simulink model "controllo_op_space"  (R2024a)
settings: Solver=VariableStepAuto  StartTime=0.0  StopTime=70  RelTol=1e-3
values from neighbouring files (symbols this model uses):
  a1 = 0.5    [avvicinamentosingolaritaforza 1.m]    (also in avvicinamentosingolaritaforza.m; cubic.m = 0; dynamicmodel.m; traiettoriafperfettadefinitiva1.m)
  a2 = 0.5    [avvicinamentosingolaritaforza 1.m]    (also in avvicinamentosingolaritaforza.m; cubic.m = 3*(s_f-s_i)/delta_t^2; dynamicmodel.m; traiettoriafperfettadefinitiva1.m)
settings Model: Creator=ACER  LastModifiedBy=UTENTE
settings OptimizationCC: ReuseModelBlockBuffer=off
settings RTWCC: GPUComputeCapability=3.5

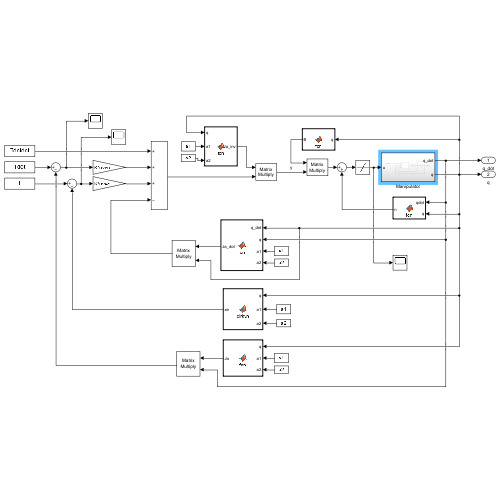
[thumbnail: Simulink's stored preview of the top-level diagram]
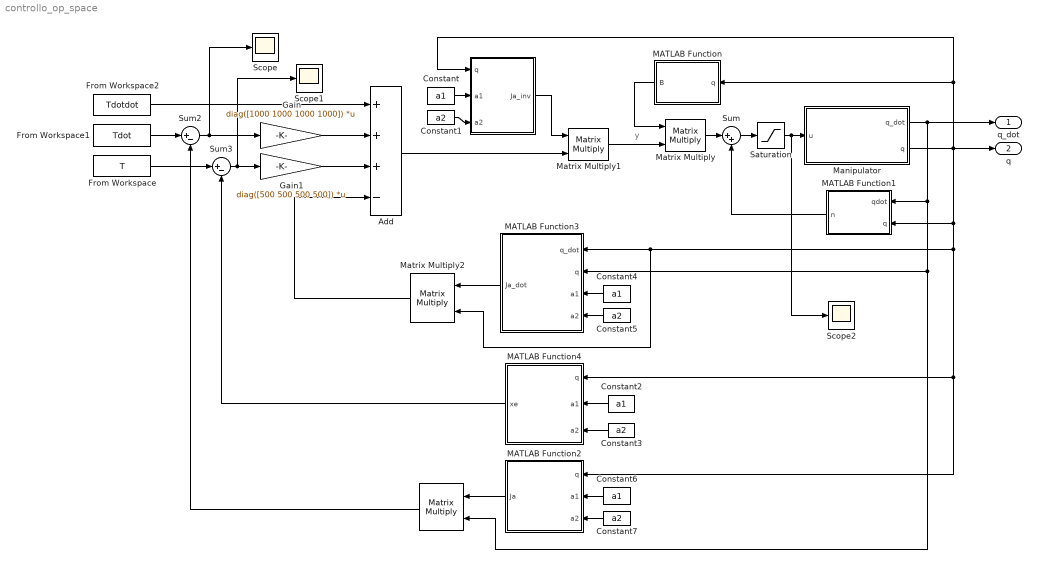
== system controllo_op_space ==
  note: y
  "  " : MATLAB Function  TreatAsAtomicUnit=on
  "   " : Product  Multiplication=Matrix(*)
  Add : Sum  Inputs=+++-
  Constant{,2,4,6} (4 alike) : Constant  Value=a1
  Constant{1,3,5,7} (4 alike) : Constant  Value=a2
  From Workspace : FromWorkspace  VariableName=T  SampleTime=0.001
  From Workspace1 : FromWorkspace  VariableName=Tdot  SampleTime=0.001
  From Workspace2 : FromWorkspace  VariableName=Tdotdot  SampleTime=0.001
  Gain : Gain  Gain=diag([1000 1000 1000 1000])  Multiplication=Matrix(K*u) (u vector)
  Gain1 : Gain  Gain=diag([500 500 500 500])  Multiplication=Matrix(K*u) (u vector)
  MATLAB Function : MATLAB Function  TreatAsAtomicUnit=on
  MATLAB Function1 : MATLAB Function  TreatAsAtomicUnit=on
  MATLAB Function2 : MATLAB Function  TreatAsAtomicUnit=on
  MATLAB Function3 : MATLAB Function  TreatAsAtomicUnit=on
  MATLAB Function4 : MATLAB Function  TreatAsAtomicUnit=on
  Manipulator : Subsystem
  Matrix Multiply : Product  Multiplication=Matrix(*)
  Matrix Multiply1 : Product  Multiplication=Matrix(*)
  Matrix Multiply2 : Product  Multiplication=Matrix(*)
  Saturation : Saturate  UpperLimit=2000  LowerLimit=-2000
  Scope : Scope
  Scope1 : Scope
  Scope2 : Scope
  Sum : Sum  Inputs=|++
  Sum2 : Sum  Inputs=|+-
  Sum3 : Sum  Inputs=|+-
  q_dot : Outport
  q : Outport  Port=2
  wires:
  MATLAB Function1/1(n) -> Sum/2
  Matrix Multiply/1 -> Sum/1
  Sum/1 -> Saturation/1
  MATLAB Function/1(B) -> Matrix Multiply/1
  Matrix Multiply1/1 -> Matrix Multiply/2
  "  "/1(Ja_inv) -> Matrix Multiply1/1
  Constant1/1 -> "  "/3(a2)
  Constant/1 -> "  "/2(a1)
  From Workspace2/1 -> Add/1
  From Workspace1/1 -> Sum2/1
  From Workspace/1 -> Sum3/1
  Sum2/1 -> Scope/1, Gain/1
  Gain/1 -> Add/2
  Sum3/1 -> Scope1/1, Gain1/1
  Gain1/1 -> Add/3
  MATLAB Function4/1(xe) -> Sum3/2
  "   "/1 -> Sum2/2
  Matrix Multiply2/1 -> Add/4
  Add/1 -> Matrix Multiply1/2
  Constant5/1 -> MATLAB Function3/4(a2)
  Constant4/1 -> MATLAB Function3/3(a1)
  Manipulator/2(q) -> q/1, MATLAB Function2/1(q), MATLAB Function4/1(q), Matrix Multiply2/2, MATLAB Function3/1(q_dot), MATLAB Function1/2(q), "  "/1(q), MATLAB Function/1(q)
  MATLAB Function3/1(Ja_dot) -> Matrix Multiply2/1
  Manipulator/1(q_dot) -> q_dot/1, "   "/2, MATLAB Function3/2(q), MATLAB Function1/1(qdot)
  MATLAB Function2/1(Ja) -> "   "/1
  Constant6/1 -> MATLAB Function2/2(a1)
  Constant7/1 -> MATLAB Function2/3(a2)
  Constant2/1 -> MATLAB Function4/2(a1)
  Constant3/1 -> MATLAB Function4/3(a2)
  Saturation/1 -> Scope2/1, Manipulator/1(u)

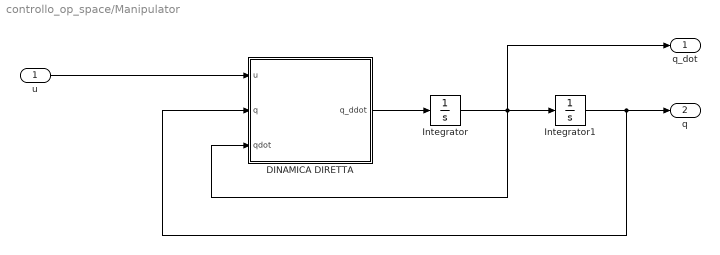
== system controllo_op_space/Manipulator ==
  u : Inport
  DINAMICA DIRETTA : MATLAB Function  TreatAsAtomicUnit=on
  Integrator : Integrator  InitialCondition=[0 0 0 0]'
  Integrator1 : Integrator  InitialCondition=[0 -pi/4 0 0]
  q_dot : Outport  VectorParamsAs1DForOutWhenUnconnected=off
  q : Outport  Port=2  VectorParamsAs1DForOutWhenUnconnected=off
  wires:
  Integrator1/1 -> q/1, DINAMICA DIRETTA/2(q)
  Integrator/1 -> q_dot/1, DINAMICA DIRETTA/3(qdot), Integrator1/1
  DINAMICA DIRETTA/1(q_ddot) -> Integrator/1
  u/1 -> DINAMICA DIRETTA/1(u)

== matlab function controllo_op_space/MATLAB Function1 ==
  data: qdot input; q input; n output
function n = fcn(qdot, q)
a1=0.5; %m
a2=0.5; %m
l1=0.25; %m
l2=0.25; %m
ml1=20; %kg
ml2=20; %kg
ml3=10; %kg
Il1=4; %kg*m^2
Il2=4; %kg*m^2
Il4=1; %kg*m^2
kr1=1;
kr2=1;
kr3=50; %rad/m
kr4 =20;
Im1=0.01; %kg*m^2
Im2=0.01; %kg*m^2
Im3=0.005; %kg*m^2
Im4=0.001; %kg*m^2
Fm1=0.00005; %N*m*s/rad
Fm2=0.00005; %N*m*s/rad
Fm3 =0.01; %N*m*s/rad
Fm4 =0.005; %N*m*s/rad
mpayload=5;

%% CALCOLO JPl JPm JOl JOm

Jp_l1=[-l1*sin(q(1)) 0 0 0;
    l1*cos(q(1)) 0 0 0;
    0 0 0 0];

Jp_l2=[-a1*sin(q(1))-l2*sin(q(1)+q(2)) -l2*sin(q(1)+q(2)) 0 0;
    a1*cos(q(1))+l2*cos(q(1)+q(2)) l2*cos(q(1)+q(2)) 0 0;
    0 0 0 0];

%poiché ml3 è nulla è inutile calcolare Jp_l3

Jp_l4=[-a1*sin(q(1))-a2*sin(q(1)+q(2)) -a2*sin(q(1)+q(2)) 0 0;
    a1*cos(q(1))+a2*cos(q(1)+q(2)) a2*cos(q(1)+q(2)) 0 0;
    0 0 -1 0];      %Jp_l4=Ja


Jo_l1=[zeros(2,4)
    1 0 0 0]; 

Jo_l2=[zeros(2,4)
    1 1 0 0];

%poiché Il3 è nullo è inutile calcolare Jo_l3

Jo_l4=[zeros(2,4)
    1 1 0 -1];       %Jo_l4=Ja;


%poiché le masse dei motori sono nulle, è inutile calcolare Jp_m 

Jo_m1=[zeros(2,4)
    kr1 0 0 0]; 

Jo_m2=[zeros(2,4)
    1 kr2 0 0];

Jo_m3=[zeros(2,4)
    1 1 kr3 0];

Jo_m4=[zeros(2,4)
    1 1 0 -kr4];  

%% CALCOLO MATRICE B (tenendo conto di braccio aumentato)
B=  ml1*(Jp_l1'*Jp_l1)+Jo_l1'*Il1*Jo_l1+Jo_m1'*Im1*Jo_m1...
    +ml2*(Jp_l2'*Jp_l2)+Jo_l2'*Il2*Jo_l2+Jo_m2'*Im2*Jo_m2...
    +Jo_m3'*Im3*Jo_m3+...
    +ml3*(Jp_l4'*Jp_l4)+Jo_l4'*Il4*Jo_l4+Jo_m4'*Im4*Jo_m4;

%% JACOBIANO DERIVATO RISPETTO A dq1 e dq2

%Jpl1 dipende solo da q1
Jpl1_dq1=[-l1*cos(q(1)) 0 0 0;
    -l1*sin(q(1)) 0 0 0;
    0 0 0 0];

Jpl2_dq1=[-a1*cos(q(1))-l2*cos(q(1)+q(2)) -l2*cos(q(1)+q(2)) 0 0;
    -a1*sin(q(1))-l2*sin(q(1)+q(2)) -l2*sin(q(1)+q(2)) 0 0;
    0 0 0 0];

Jpl2_dq2=[-a2*cos(q(1)+q(2)) -a2*cos(q(1)+q(2)) 0 0;
    -a2*sin(q(1)+q(2)) -a2*sin(q(1)+q(2)) 0 0;
    0 0 0 0];

Jpl4_dq1=[-a1*cos(q(1))-a2*cos(q(1)+q(2)) -a2*cos(q(1)+q(2)) 0 0;
    -a1*sin(q(1))-a2*sin(q(1)+q(2)) -a2*sin(q(1)+q(2)) 0 0;
    0 0 0 0];

Jpl4_dq2=[-a2*sin(q(1)+q(2)) -a2*sin(q(1)+q(2)) 0 0;
    -a2*cos(q(1)+q(2)) -a2*cos(q(1)+q(2)) 0 0;
    0 0 0 0];

%i Jo non dipendono da nessuna q

%% Calcolo matrice differenziate rispetto a dq1 dq2
dBdq1=ml1*(Jpl1_dq1'*Jp_l1+Jp_l1'*Jpl1_dq1)+ml2*(Jpl2_dq1'*Jp_l2+Jp_l2'*Jpl2_dq1)...
    +ml3*(Jpl4_dq1'*Jp_l4+Jp_l4'*Jpl4_dq1);
dBdq2=ml2*(Jpl2_dq2'*Jp_l2+Jp_l2'*Jpl2_dq2)+ml3*(Jpl4_dq2'*Jp_l4+Jp_l4'*Jpl4_dq2);

%B non dipende da q3 e q4

H=zeros(4,4,4);

%% Inizializzazione simboli cristoffel del primo tipo
for i=1:4
    for j=1:4
        for k=1:4
            H(i,j,k)=0;
        end
    end
end

%ricordiamo che B è simmetrica quindi hijk=hikj
%inoltre tutti i hiii sono nulli

H(1,1,2)=1/2*(dBdq2(1,1)+dBdq1(1,2)-dBdq1(1,2));
H(1,2,1)=H(1,1,2); %per simmetria
H(1,2,2)=1/2*(dBdq2(1,2)+dBdq2(1,2)-dBdq1(2,2));
H(2,1,1)=1/2*(dBdq1(2,1)+dBdq1(2,1)-dBdq2(1,1));
H(2,1,2)=1/2*(dBdq2(2,1)+dBdq1(2,2)-dBdq2(1,2));
H(2,2,1)=H(2,1,2); %per simmetria
H(2,2,2)=1/2*(dBdq2(2,2)+dBdq2(2,2)-dBdq2(2,2));

%non calcoliamo H3 H4 perchè la terza e quarta riga di dB sono nulle

% C=sym('C',[4,4]);
C=zeros(4,4);
for i=1:4
    for j=1:4
        C(i,j)=0;
    end
end

% qdot=sym('qdot',[4,1]);

for i=1:4
    for j=1:4
        %qui ho il generico Cij dato dalla somma su k di cijk*qk_dot
        for k=1:4
            r=H(i,j,k)*qdot(k);
            C(i,j)=C(i,j)+r;
        end
    end
end

% qdotdot=sym('qdotdot',[4 1]);

g=[0 0 -9.81*(ml3+mpayload) 0]';

Fv=diag([kr1^2*Fm1 kr2^2*Fm2 kr3^2*Fm3 kr4^2*Fm4]);


 n=C*qdot+Fv*qdot+g;

end

== matlab function controllo_op_space/MATLAB Function ==
  data: q input; B output
function B = fcn(q)
a1=0.5; %m
a2=0.5; %m
l1=0.25; %m
l2=0.25; %m
ml1=20; %kg
ml2=20; %kg
ml3=10; %kg
Il1=4; %kg*m^2
Il2=4; %kg*m^2
Il4=1; %kg*m^2
kr1=1;
kr2=1;
kr3=50; %rad/m
kr4 =20;
Im1=0.01; %kg*m^2
Im2=0.01; %kg*m^2
Im3=0.005; %kg*m^2
Im4=0.001; %kg*m^2

%% CALCOLO JPl JPm JOl JOm

Jp_l1=[-l1*sin(q(1)) 0 0 0;
    l1*cos(q(1)) 0 0 0;
    0 0 0 0];

Jp_l2=[-a1*sin(q(1))-l2*sin(q(1)+q(2)) -l2*sin(q(1)+q(2)) 0 0;
    a1*cos(q(1))+l2*cos(q(1)+q(2)) l2*cos(q(1)+q(2)) 0 0;
    0 0 0 0];

%poiché ml3 è nulla è inutile calcolare Jp_l3

Jp_l4=[-a1*sin(q(1))-a2*sin(q(1)+q(2)) -a2*sin(q(1)+q(2)) 0 0;
    a1*cos(q(1))+a2*cos(q(1)+q(2)) a2*cos(q(1)+q(2)) 0 0;
    0 0 -1 0];      %Jp_l4=Ja


Jo_l1=[zeros(2,4)
    1 0 0 0]; 

Jo_l2=[zeros(2,4)
    1 1 0 0];

%poiché Il3 è nullo è inutile calcolare Jo_l3

Jo_l4=[zeros(2,4)
    1 1 0 -1];       %Jo_l4=Ja;


%poiché le masse dei motori sono nulle, è inutile calcolare Jp_m 

Jo_m1=[zeros(2,4)
    kr1 0 0 0]; 

Jo_m2=[zeros(2,4)
    1 kr2 0 0];

Jo_m3=[zeros(2,4)
    1 1 kr3 0];

Jo_m4=[zeros(2,4)
    1 1 0 -kr4];  

%% CALCOLO MATRICE B (tenendo conto di braccio aumentato)
B=  ml1*(Jp_l1'*Jp_l1)+Jo_l1'*Il1*Jo_l1+Jo_m1'*Im1*Jo_m1...
    +ml2*(Jp_l2'*Jp_l2)+Jo_l2'*Il2*Jo_l2+Jo_m2'*Im2*Jo_m2...
    +Jo_m3'*Im3*Jo_m3+...
    +ml3*(Jp_l4'*Jp_l4)+Jo_l4'*Il4*Jo_l4+Jo_m4'*Im4*Jo_m4;

== matlab function controllo_op_space/Manipulator/DINAMICA DIRETTA ==
  data: u input; q_ddot output; q input; qdot input
function q_ddot = fcn(u, q, qdot)

d0=1; %m
a1=0.5; %m
a2=0.5; %m
l1=0.25; %m
l2=0.25; %m
ml1=20; %kg
ml2=20; %kg
ml3=10; %kg
Il1=4; %kg*m^2
Il2=4; %kg*m^2
Il4=1; %kg*m^2
kr1=1;
kr2=1;
kr3=50; %rad/m
kr4 =20;
Im1=0.01; %kg*m^2
Im2=0.01; %kg*m^2
Im3=0.005; %kg*m^2
Im4=0.001; %kg*m^2
Fm1=0.00005; %N*m*s/rad
Fm2=0.00005; %N*m*s/rad
Fm3 =0.01; %N*m*s/rad
Fm4 =0.005; %N*m*s/rad
mpayload=5;

%% CALCOLO JPl JPm JOl JOm

Jp_l1=[-l1*sin(q(1)) 0 0 0;
    l1*cos(q(1)) 0 0 0;
    0 0 0 0];

Jp_l2=[-a1*sin(q(1))-l2*sin(q(1)+q(2)) -l2*sin(q(1)+q(2)) 0 0;
    a1*cos(q(1))+l2*cos(q(1)+q(2)) l2*cos(q(1)+q(2)) 0 0;
    0 0 0 0];

%poiché ml3 è nulla è inutile calcolare Jp_l3

Jp_l4=[-a1*sin(q(1))-a2*sin(q(1)+q(2)) -a2*sin(q(1)+q(2)) 0 0;
    a1*cos(q(1))+a2*cos(q(1)+q(2)) a2*cos(q(1)+q(2)) 0 0;
    0 0 -1 0];      %Jp_l4=Ja


Jo_l1=[zeros(2,4)
    1 0 0 0]; 

Jo_l2=[zeros(2,4)
    1 1 0 0];

%poiché Il3 è nullo è inutile calcolare Jo_l3

Jo_l4=[zeros(2,4)
    1 1 0 -1];       %Jo_l4=Ja;


%poiché le masse dei motori sono nulle, è inutile calcolare Jp_m 

Jo_m1=[zeros(2,4)
    kr1 0 0 0]; 

Jo_m2=[zeros(2,4)
    1 kr2 0 0];

Jo_m3=[zeros(2,4)
    1 1 kr3 0];

Jo_m4=[zeros(2,4)
    1 1 0 -kr4];  

%% CALCOLO MATRICE B (tenendo conto di braccio aumentato)
B=  ml1*(Jp_l1'*Jp_l1)+Jo_l1'*Il1*Jo_l1+Jo_m1'*Im1*Jo_m1...
    +ml2*(Jp_l2'*Jp_l2)+Jo_l2'*Il2*Jo_l2+Jo_m2'*Im2*Jo_m2...
    +Jo_m3'*Im3*Jo_m3+...
    +ml3*(Jp_l4'*Jp_l4)+Jo_l4'*Il4*Jo_l4+Jo_m4'*Im4*Jo_m4;

%% JACOBIANO DERIVATO RISPETTO A dq1 e dq2

%Jpl1 dipende solo da q1
Jpl1_dq1=[-l1*cos(q(1)) 0 0 0;
    -l1*sin(q(1)) 0 0 0;
    0 0 0 0];

Jpl2_dq1=[-a1*cos(q(1))-l2*cos(q(1)+q(2)) -l2*cos(q(1)+q(2)) 0 0;
    -a1*sin(q(1))-l2*sin(q(1)+q(2)) -l2*sin(q(1)+q(2)) 0 0;
    0 0 0 0];

Jpl2_dq2=[-a2*cos(q(1)+q(2)) -a2*cos(q(1)+q(2)) 0 0;
    -a2*sin(q(1)+q(2)) -a2*sin(q(1)+q(2)) 0 0;
    0 0 0 0];

Jpl4_dq1=[-a1*cos(q(1))-a2*cos(q(1)+q(2)) -a2*cos(q(1)+q(2)) 0 0;
    -a1*sin(q(1))-a2*sin(q(1)+q(2)) -a2*sin(q(1)+q(2)) 0 0;
    0 0 0 0];

Jpl4_dq2=[-a2*sin(q(1)+q(2)) -a2*sin(q(1)+q(2)) 0 0;
    -a2*cos(q(1)+q(2)) -a2*cos(q(1)+q(2)) 0 0;
    0 0 0 0];

%i Jo non dipendono da nessuna q

%% Calcolo matrice differenziate rispetto a dq1 dq2
dBdq1=ml1*(Jpl1_dq1'*Jp_l1+Jp_l1'*Jpl1_dq1)+ml2*(Jpl2_dq1'*Jp_l2+Jp_l2'*Jpl2_dq1)...
    +ml3*(Jpl4_dq1'*Jp_l4+Jp_l4'*Jpl4_dq1);
dBdq2=ml2*(Jpl2_dq2'*Jp_l2+Jp_l2'*Jpl2_dq2)+ml3*(Jpl4_dq2'*Jp_l4+Jp_l4'*Jpl4_dq2);

%B non dipende da q3 e q4

H=zeros(4,4,4);

%% Inizializzazione simboli cristoffel del primo tipo
for i=1:4
    for j=1:4
        for k=1:4
            H(i,j,k)=0;
        end
    end
end

%ricordiamo che B è simmetrica quindi hijk=hikj
%inoltre tutti i hiii sono nulli

H(1,1,2)=1/2*(dBdq2(1,1)+dBdq1(1,2)-dBdq1(1,2));
H(1,2,1)=H(1,1,2); %per simmetria
H(1,2,2)=1/2*(dBdq2(1,2)+dBdq2(1,2)-dBdq1(2,2));
H(2,1,1)=1/2*(dBdq1(2,1)+dBdq1(2,1)-dBdq2(1,1));
H(2,1,2)=1/2*(dBdq2(2,1)+dBdq1(2,2)-dBdq2(1,2));
H(2,2,1)=H(2,1,2); %per simmetria
H(2,2,2)=1/2*(dBdq2(2,2)+dBdq2(2,2)-dBdq2(2,2));

%non calcoliamo H3 H4 perchè la terza e quarta riga di dB sono nulle

% C=sym('C',[4,4]);
C=zeros(4,4);
for i=1:4
    for j=1:4
        C(i,j)=0;
    end
end

% qdot=sym('qdot',[4,1]);

for i=1:4
    for j=1:4
        %qui ho il generico Cij dato dalla somma su k di cijk*qk_dot
        for k=1:4
            r=H(i,j,k)*qdot(k);
            C(i,j)=C(i,j)+r;
        end
    end
end

% qdotdot=sym('qdotdot',[4 1]);

g=[0 0 -9.81*(ml3+mpayload) 0]';

Fv=diag([kr1^2*Fm1 kr2^2*Fm2 kr3^2*Fm3 kr4^2*Fm4]);

%% qdotdot=inv(B)(tau-tau_primo)

 q_ddot=inv(B)*(u-C*qdot-Fv*qdot-g);

end

== matlab function controllo_op_space/   ==
  data: q input; Ja_inv output; a1 input; a2 input
function Ja_inv = fcn(q, a1, a2)

Ja=[-a1*sin(q(1))-a2*sin(q(1)+q(2)), -a2*sin(q(1)+q(2)), 0, 0;
    a1*cos(q(1))+ a2*cos(q(1)+q(2)), a2*cos(q(1)+q(2)), 0, 0;
    0, 0, -1, 0;
    1, 1, 0, -1];
Ja_inversa=inv(Ja);
Ja_inv = Ja_inversa;

== matlab function controllo_op_space/MATLAB Function4 ==
  data: q input; xe output; a1 input; a2 input
function xe = dirkyn(q, a1, a2)

xe=[a1*cos(q(1))+ a2*cos(q(1)+q(2));
    a1*sin(q(1))+ a2*sin(q(1)+q(2));
    1-q(3);
    q(1)+q(2)-q(4)];

== matlab function controllo_op_space/MATLAB Function3 ==
  data: q_dot input; q input; Ja_dot output; a1 input; a2 input
function Ja_dot = fcn(q_dot, q, a1, a2)

Ja_dot= [ q_dot(1)*(-a1*cos(q(1))-a2*cos(q(1)+q(2))), q_dot(2)*(-a2*cos(q(1)+q(2))), 0, 0;
          q_dot(1)*(-a1*sin(q(1))-a2*sin(q(1)+q(2))), q_dot(2)*(-a2*sin(q(1)+q(2))), 0, 0;
         0 0 0 0;
         0 0 0 0];

== matlab function controllo_op_space/MATLAB Function2 ==
  data: q input; Ja output; a1 input; a2 input
function Ja = fcn(q, a1, a2)

Ja=[-a1*sin(q(1))-a2*sin(q(1)+q(2)), -a2*sin(q(1)+q(2)), 0, 0;
    a1*cos(q(1))+ a2*cos(q(1)+q(2)), a2*cos(q(1)+q(2)), 0, 0;
    0, 0, -1, 0;
    1, 1, 0, -1];
